simulink model "etherCATmdl2"  (R2022a)
settings: Solver=FixedStepDiscrete  StartTime=0.0  StopTime=inf  RelTol=1e-3
PreLoadFcn:
  | Ts_IO133 = 0.001;
  | Ts_IO750 = 0.001;
InitFcn:
  | Ts_IO133 = 0.001
StopFcn:
  | if isfile(['sdi_view_',bdroot,'.mldatx'])
  |  Simulink.sdi.clearPreferences();
  |  Simulink.sdi.view();
  |  pause(3);
  |  Simulink.sdi.loadView(['sdi_view_',bdroot,]);
  | end
undefined symbols (not defined in the file or in its folder): AUS0, AUS1, C, CAN, FD, padding, Statuswort, Steuerwort
libraries: speedgoatlib_IO602 x9, slrealtimeutilitieslib x8, speedgoatlib_IO133 x5, speedgoatlib_IO750 x5, canfdmsglib x4, canmsglib x4, etargetslib x2, slrealtimeloglib x2, simulink x1
settings Model: SimulationMode=external  ExtModeEnableFloating=off  Creator=sandro.reichenbach  LastModifiedBy=muhammet.cingoez
settings SolverCC: ConcurrentTasks=on  PositivePriorityOrder=on
settings DataIOCC: LimitDataPoints=on  SaveFormat=StructureWithTime
settings OptimizationCC: BlockReduction=off  OptimizeBlockIOStorage=off
settings DebuggingCC: TasksWithSamePriorityMsg=none
settings HardwareCC: ProdBitPerLong=64  ProdLongLongMode=on  ProdHWDeviceType=Intel->x86-64 (Linux 64)
settings RTWCC: Description=Simulink Real-Time  SystemTargetFile=slrealtime.tlc  TemplateMakefile=slrealtime_default_tmf  RTWVerbose=off  Toolchain=Simulink Real-Time Toolchain  BuildConfiguration=Faster Runs  CodeExecutionProfiling=on  TargetLang=C++  DLArmComputeVersion=19.05

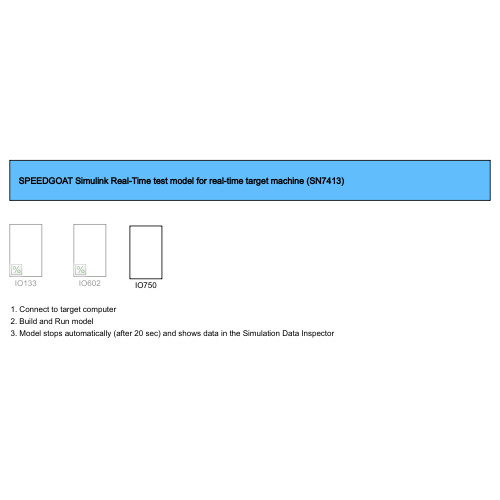
[thumbnail: Simulink's stored preview of the top-level diagram]
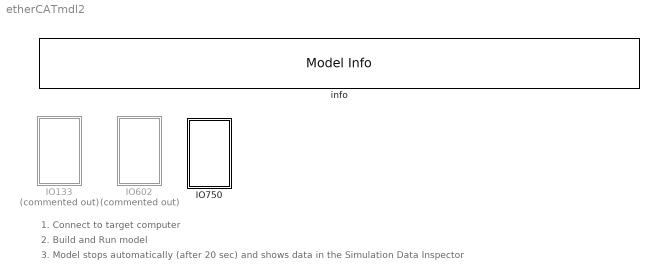
== system etherCATmdl2 ==
  note: 1. Connect to target computer
  note: 2. Build and Run model
  note: 3. Model stops automatically (after 20 sec) and shows data in the Simulation Data Inspector
  IO133 : Subsystem  Commented=on
  IO602 : Subsystem  Commented=on
  IO750 : Subsystem
  info : simulink/Model-Wide Utilities/Model Info  Frame=on  DisplayStringWithTags=SPEEDGOAT Simulink Real-Time test model for real-time target machine (SN7413)  HorizontalTextAlignment=Left  LeftAlignmentValue=0.02

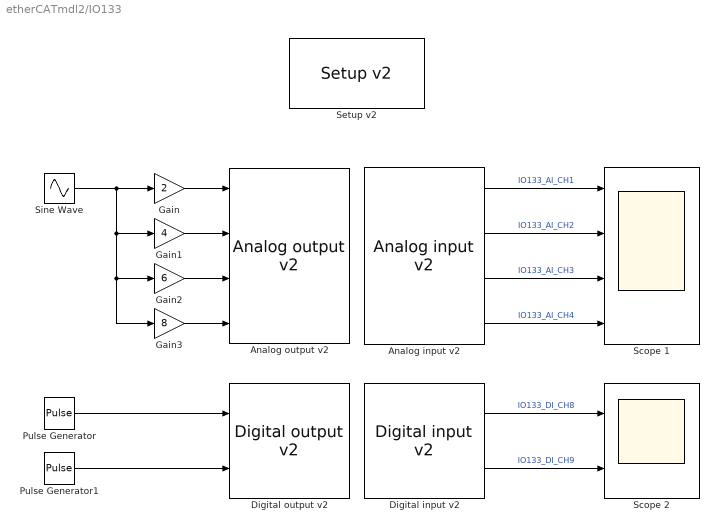
== system etherCATmdl2/IO133 ==
  "Analog input v2 " : speedgoatlib_IO133/Analog input v2   parModuleId=1  parSampleTime=Ts_IO133  parPciSlot=-1  parAdcChannels=[1 2 3 4]  parAdcVoltageRange=[2 2]  parAdcOversamplRate=[1 1]  parAdcContSampling=0  parAdcDmaEnable=0  parAdcActiveDmaDevices=[1 1]  parAdcFrameSize=100
      settings: SourceProductName=Simulink Real-Time: Speedgoat I/O Driver Library
  "Analog output v2 " : speedgoatlib_IO133/Analog output v2   parModuleId=1  parSampleTime=Ts_IO133  parPciSlot=-1  parDacChannels=[1 2 3 4]  parDacVoltageRange=[4 4 6 6 5 5 5 5]  parDacInitValues=[0 0 0 0]  parDacReset=[1 1 1 1]  parDacSyncOut=1  parDacDmaEnable=0  parDacActiveDmaDevices=[1 1]  parDacDmaLatency=2  parDacFrameSize=100
      settings: SourceProductName=Simulink Real-Time: Speedgoat I/O Driver Library
  "Digital input v2 " : speedgoatlib_IO133/Digital input v2   parModuleId=1  parSampleTime=Ts_IO133  parPciSlot=-1  parDiChannels=[8 9]
      settings: SourceProductName=Simulink Real-Time: Speedgoat I/O Driver Library
  "Digital output v2 " : speedgoatlib_IO133/Digital output v2   parModuleId=1  parSampleTime=Ts_IO133  parPciSlot=-1  parDoChannels=[1 2]  parDoInitValues=[0 0]  parDoReset=[1 1]
      settings: SourceProductName=Simulink Real-Time: Speedgoat I/O Driver Library
  Gain : Gain  Gain=2
  Gain1 : Gain  Gain=4
  Gain2 : Gain  Gain=6
  Gain3 : Gain  Gain=8
  Pulse Generator : DiscretePulseGenerator  Period=20  PulseWidth=5  SampleTime=-1
  Pulse Generator1 : DiscretePulseGenerator  Period=20  PulseWidth=10  SampleTime=-1
  Scope 1 : Scope  NumInputPorts=4
  Scope 2 : Scope  NumInputPorts=2
  "Setup v2 " : speedgoatlib_IO133/Setup v2   parPciSlot=-1  parModuleId=1  parInterModuleSync=None  parConvClockBaseRate=20MHz  parConvClock1Divider=20000  parConvClock2Divider=20000  parFrameTriggerEnable=off  parFrameTriggerDivider=10  parConvClock1BaseRate=1  parConvClock2BaseRate=1  parFrameTriggerClock=1  parAdcChannels=1:4  parAdcRange1=+-10V  parAdcRange2=+-10V  parAdcVoltageRange=[2 2]  parAdcOversampling1=None  parAdcOversampling2=None  parAdcOversamplRate=[1 1]  parAdcAutoCorrection=on  parAdcContSampling=off  parAdcDmaEnable=off  parAdcDmaClock=Clock 1  parAdcFrameSize_=100  parAdcSampleTime_=-1  parAdcActiveDmaDevices=[1 1]  parAdcFrameTriggerEnable=0  parAdcFrameSize=100  parAdcSampleTime=0.1  parDacChannels=1:4  parDacInitValues=0  parDacReset=1  parDacRange1=+-5V  parDacRange2=+-5V  parDacRange3=+-10.8V  parDacRange4=+-10.8V  parDacRange5=+-10V  parDacRange6=+-10V  parDacRange7=+-10V  parDacRange8=+-10V  parDacVoltageRange=[4 4 6 6 5 5 5 5]  parDacAutoCorrection=on  parDacSyncOut=on  parDacDmaEnable=off  parDacDmaLatency=Until next frame  parDacDmaClock=Clock 1  parDacFrameSize_=100  parDacSampleTime_=-1  parDacActiveDmaDevices=[1 1]  parDacFrameTriggerEnable=0  parDacFrameSize=100  parDacSampleTime=0.1  parDoChannels=1:2  parDoInitValues=0  parDoReset=1  parDiChannels=8:9  parDiDebounceEnable=off  parDiDebounceTime=0  parDiDebounceValue=0  parDioPullRefFront=Pull-up 3.3V  parDioPullRefRear=Floating
      settings: SourceProductName=Simulink Real-Time: Speedgoat I/O Driver Library
  Sine Wave : Sin  Frequency=50  SampleTime=0
  wires:
  Pulse Generator/1 -> "Digital output v2 "/1
  Gain1/1 -> "Analog output v2 "/2
  Gain/1 -> "Analog output v2 "/1
  Gain3/1 -> "Analog output v2 "/4
  Gain2/1 -> "Analog output v2 "/3
  Sine Wave/1 -> Gain/1, Gain1/1, Gain2/1, Gain3/1
  Pulse Generator1/1 -> "Digital output v2 "/2
  "Analog input v2 "/1 -> Scope 1/1  "IO133_AI_CH1"
  "Analog input v2 "/2 -> Scope 1/2  "IO133_AI_CH2"
  "Analog input v2 "/3 -> Scope 1/3  "IO133_AI_CH3"
  "Analog input v2 "/4 -> Scope 1/4  "IO133_AI_CH4"
  "Digital input v2 "/1 -> Scope 2/1  "IO133_DI_CH8"
  "Digital input v2 "/2 -> Scope 2/2  "IO133_DI_CH9"

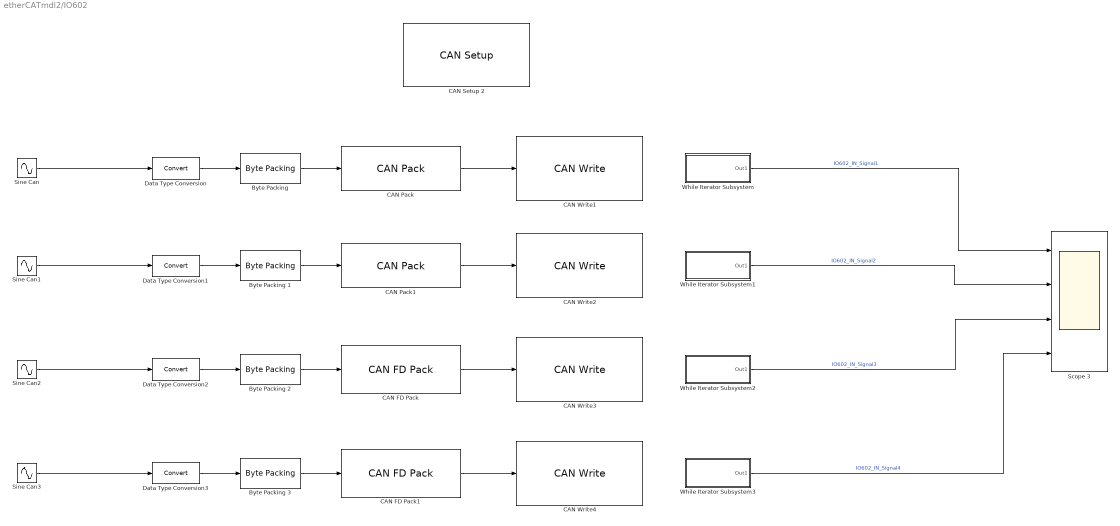
== system etherCATmdl2/IO602 ==
  Byte Packing {,1..3} (4 alike) : slrealtimeutilitieslib/Byte Packing  MaskPackedDataType=uint8  MaskUnpackedDataTypes={'single'}  MaskAlignment=1
  CAN FD Pack : canfdmsglib/CAN FD Pack  MsgList=(none)  MsgName=Msg  ProtocolMode=CAN FD  MsgIDType=Standard (11-bit identifier)  MsgIdentifier=102  MsgLength=4  Remote=off  BRSSwitch=off  ApplyMinMax=off  SignalInfo={}
      settings: SourceProductBaseCode=XP,ME,VN  DataFormat=raw data
  CAN FD Pack1 : canfdmsglib/CAN FD Pack  MsgList=(none)  MsgName=Msg  ProtocolMode=CAN FD  MsgIDType=Standard (11-bit identifier)  MsgIdentifier=103  MsgLength=4  Remote=off  BRSSwitch=off  ApplyMinMax=off  SignalInfo={}
      settings: SourceProductBaseCode=XP,ME,VN  DataFormat=raw data
  CAN Pack : canmsglib/CAN Pack  MsgList=(none)  MsgName=CAN Msg  MsgIDType=Standard (11-bit identifier)  MsgIdentifier=100  MsgLength=4  Remote=off  ApplyMinMax=off  BusOutput=off  SignalInfo={}
      settings: SourceProductBaseCode=XP,ME,VN  DataFormat=raw data
  CAN Pack1 : canmsglib/CAN Pack  MsgList=(none)  MsgName=CAN Msg  MsgIDType=Standard (11-bit identifier)  MsgIdentifier=101  MsgLength=4  Remote=off  ApplyMinMax=off  BusOutput=off  SignalInfo={}
      settings: SourceProductBaseCode=XP,ME,VN  DataFormat=raw data
  CAN Setup 2 : speedgoatlib_IO602/Legacy/CAN Setup   moduletype=IO602  id=1  pciSlot=-1  chn1=CAN (HS)  chn2=CAN (HS)  chn3=CAN-FD  chn4=CAN-FD  initStruct=[]  termStruct=[]  ArbitrationbdrChn1=1.0 MBaud  ArbitrationManbdrChn1=[2,8,31,8]  FdbdrChn1=5.0 MBaud  FdManbdrChn1=[2,2,5,2]  ArbitrationbdrChn2=1.0 MBaud  ArbitrationManbdrChn2=[2,8,31,8]  FdbdrChn2=5.0 MBaud  FdManbdrChn2=[2,2,5,2]  ArbitrationbdrChn3=1.0 MBaud  ArbitrationManbdrChn3=[2,8,31,8]  FdbdrChn3=5.0 MBaud  FdManbdrChn3=[2,2,5,2]  ArbitrationbdrChn4=1.0 MBaud  ArbitrationManbdrChn4=[2,8,31,8]  FdbdrChn4=5.0 MBaud  FdManbdrChn4=[2,2,5,2]  moduleInitValues=[602 1 -1 -1]
      settings: SourceProductName=Simulink Real-Time: Speedgoat I/O Blockset
  CAN Write1 : speedgoatlib_IO602/Legacy/CAN Write  id=1  ts=-1  channel=1  messageType=CAN  BusInput=off  enableStatusPort=off  canType=CAN (HS)  initValues=[602 1 -1 0 1 1 0 0]
      settings: SourceProductName=Simulink Real-Time: Speedgoat I/O Blockset
  CAN Write2 : speedgoatlib_IO602/Legacy/CAN Write  id=1  ts=-1  channel=2  messageType=CAN  BusInput=off  enableStatusPort=off  canType=CAN (HS)  initValues=[602 1 -1 1 1 1 0 0]
      settings: SourceProductName=Simulink Real-Time: Speedgoat I/O Blockset
  CAN Write3 : speedgoatlib_IO602/Legacy/CAN Write  id=1  ts=-1  channel=3  messageType=CAN  BusInput=off  enableStatusPort=off  canType=CAN-FD  initValues=[602 1 -1 2 1 2 0 0]
      settings: SourceProductName=Simulink Real-Time: Speedgoat I/O Blockset
  CAN Write4 : speedgoatlib_IO602/Legacy/CAN Write  id=1  ts=-1  channel=4  messageType=CAN  BusInput=off  enableStatusPort=off  canType=CAN-FD  initValues=[602 1 -1 3 1 2 0 0]
      settings: SourceProductName=Simulink Real-Time: Speedgoat I/O Blockset
  Data Type Conversion{,1..3} (4 alike) : DataTypeConversion  SaturateOnIntegerOverflow=off  RndMeth=Floor
  Scope 3 : Scope  NumInputPorts=4
  Sine Can : Sin  Amplitude=50  Frequency=10*2*pi  SampleTime=0.005
  Sine Can1 : Sin  Amplitude=20  Frequency=10*2*pi  SampleTime=0.005
  Sine Can2 : Sin  Amplitude=30  Frequency=10*2*pi  SampleTime=0.005
  Sine Can3 : Sin  Amplitude=40  Frequency=10*2*pi  SampleTime=0.005
  While Iterator Subsystem : Subsystem  TreatAsAtomicUnit=on
  While Iterator Subsystem1 : Subsystem  TreatAsAtomicUnit=on
  While Iterator Subsystem2 : Subsystem  TreatAsAtomicUnit=on
  While Iterator Subsystem3 : Subsystem  TreatAsAtomicUnit=on
  wires:
  While Iterator Subsystem/1(Out1) -> Scope 3/1  "IO602_IN_Signal1"
  Data Type Conversion/1 -> "Byte Packing "/1
  Sine Can/1 -> Data Type Conversion/1
  CAN Pack/1 -> CAN Write1/1
  "Byte Packing "/1 -> CAN Pack/1
  Byte Packing 1/1 -> CAN Pack1/1
  CAN Pack1/1 -> CAN Write2/1
  Sine Can1/1 -> Data Type Conversion1/1
  Data Type Conversion1/1 -> Byte Packing 1/1
  While Iterator Subsystem1/1(Out1) -> Scope 3/2  "IO602_IN_Signal2"
  While Iterator Subsystem3/1(Out1) -> Scope 3/4  "IO602_IN_Signal4"
  Data Type Conversion3/1 -> Byte Packing 3/1
  Sine Can3/1 -> Data Type Conversion3/1
  CAN FD Pack1/1 -> CAN Write4/1
  Byte Packing 3/1 -> CAN FD Pack1/1
  Byte Packing 2/1 -> CAN FD Pack/1
  CAN FD Pack/1 -> CAN Write3/1
  Sine Can2/1 -> Data Type Conversion2/1
  Data Type Conversion2/1 -> Byte Packing 2/1
  While Iterator Subsystem2/1(Out1) -> Scope 3/3  "IO602_IN_Signal3"

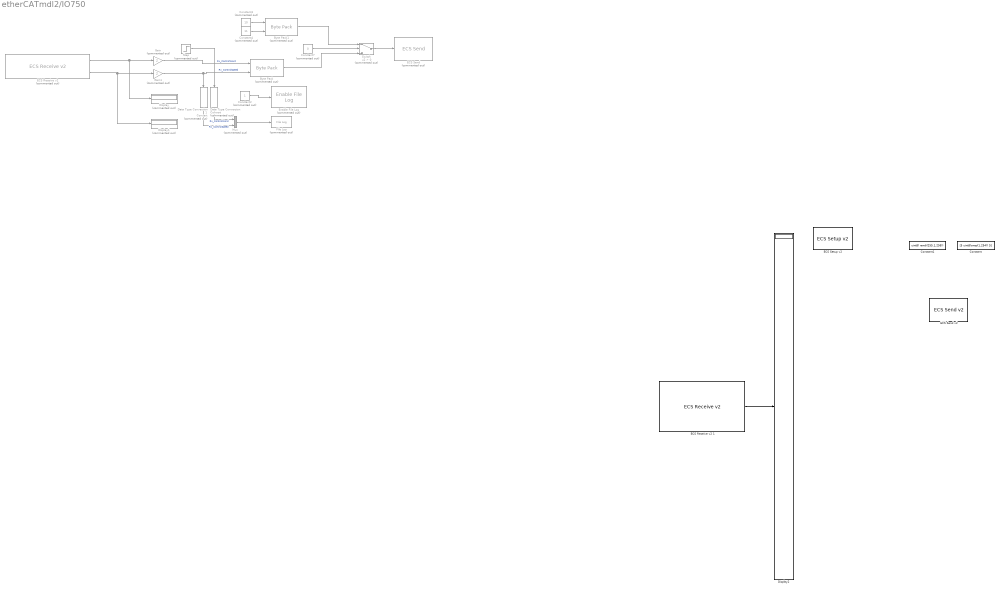
== system etherCATmdl2/IO750 ==
  Byte Pack : etargetslib/Byte Pack  Commented=on  datatypes={'uint32','single'}  byteAlign=1
  Byte Pack1 : etargetslib/Byte Pack  Commented=on  datatypes={'uint32','single'}  byteAlign=1
  Constant : Constant  Value=[5 uint8(ones(1,254)) 5]
  Constant1 : Constant  Value=uint8( randi(255,1,256))
  Constant2 : Constant  Commented=on  OutDataTypeStr=boolean
  Constant3 : Constant  Commented=on  Value=10  OutDataTypeStr=uint32
  Constant4 : Constant  Commented=on  Value=11  OutDataTypeStr=single
  Constant7 : Constant  Commented=on  Value=0  OutDataTypeStr=boolean
  Data Type Conversion : DataTypeConversion  Commented=on  SaturateOnIntegerOverflow=off  RndMeth=Floor
  Data Type Conversion1 : DataTypeConversion  Commented=on  SaturateOnIntegerOverflow=off  RndMeth=Floor
  Display : Display  Commented=on
  Display1 : Display  Commented=on
  Display2 : Display
  "ECS Receive v2 " : speedgoatlib_IO750/ECS Receive v2   Commented=on  id=1  portType=Separate signals  sampleTime=Ts_IO750  pdoTable={ 'Rx', 'ControlWord', 'uint32'; 'Rx', 'ControlSpeed', 'single' }
      settings: SourceProductName=Simulink Real-Time: Speedgoat I/O Blockset
  ECS Receive v2 1 : speedgoatlib_IO750/ECS Receive v2   id=1  portType=Byte vector  sampleTime=Ts_IO750  pdoTable={'Rx1','myvar1','uint8';'Rx2','myvar2','uint8';'Rx3','myvar3','uint8';'Rx4','myvar4','uint8';'Rx5','myvar5','uint8';'Rx6','myvar6','uint8';'Rx7','myvar7','uint8';'Rx8','myvar8','uint8';'Rx9','myvar9','uint8';'Rx10','myvar10','uint8';'Rx11','myvar11','uint8';'Rx12','myvar12','uint8';'Rx13','myvar13','uint8';'Rx14','myvar14','uint8';'Rx15','myvar15','uint8';'Rx16','myvar16','uint8';'Rx17','myvar17','uint8';'Rx18','myvar18','uint8';'Rx19','myvar19','uint8';'Rx20','myvar20','uint8';'Rx21','myvar21','uint8';'Rx22','myvar22','uint8';'Rx23','myvar23','uint8';'Rx24','myvar24','uint8';'Rx25','myvar25','uint8';'Rx26','myvar26','uint8';'Rx27','myvar27','uint8';'Rx28','myvar28','uint8';'Rx29','myvar29','uint8';'Rx30','myvar30','uint8';'Rx31','myvar31','uint8';'Rx32','myvar32','uint8';'Rx33','myvar33','uint8';'Rx34','myvar34','uint8';'Rx35','myvar35','uint8';'Rx36','myvar36','uint8';'Rx37','myvar37','uint8';'Rx38','myvar38','uint8';'Rx39','myvar39','uint8';'Rx40','myvar40','uint8';'Rx41','myvar41','uint8';'Rx42','myvar42','uint8';'Rx43','myvar43','uint8';'Rx44','myvar44','uint8';'Rx45','myvar45','uint8';'Rx46','myvar46','uint8';'Rx47','myvar47','uint8';'Rx48','myvar48','uint8';'Rx49','myvar49','uint8';'Rx50','myvar50','uint8';'Rx51','myvar51','uint8';'Rx52','myvar52','uint8';'Rx53','myvar53','uint8';'Rx54','myvar54','uint8';'Rx55','myvar55','uint8';'Rx56','myvar56','uint8';'Rx57','myvar57','uint8';'Rx58','myvar58','uint8';'Rx59','myvar59','uint8';'Rx60','myvar60','uint8';'Rx61','myvar61','uint8';'Rx62','myvar62','uint8';'Rx63','myvar63','uint8';'Rx64','myvar64','uint8';'Rx65','myvar65','uint8';'Rx66','myvar66','uint8';'Rx67','myvar67','uint8';'Rx68','myvar68','uint8';'Rx69','myvar69','uint8';'Rx70','myvar70','uint8';'Rx71','myvar71','uint8';'Rx72','myvar72','uint8';'Rx73','myvar73','uint8';'Rx74','myvar74','uint8';'Rx75','myvar75','uint8';'Rx76','myvar76','uint8';'Rx77','myvar77','uint8';'Rx78','myvar78','uint8';'Rx79','myvar79','uint8';'Rx80','myvar80','uint8';'Rx81','myvar81','uint8';'Rx82','myvar82','uint8';'Rx83','myvar83','uint8';'Rx84','myvar84','uint8';'Rx85','myvar85','uint8';'Rx86','myvar86','uint8';'Rx87','myvar87','uint8';'Rx88','myvar88','uint8';'Rx89','myvar89','uint8';'Rx90','myvar90','uint8';'Rx91','myvar91','uint8';'Rx92','myvar92','uint8';'Rx93','myvar93','uint8';'Rx94','myvar94','uint8';'Rx95','myvar95','uint8';'Rx96','myvar96','uint8';'Rx97','myvar97','uint8';'Rx98','myvar98','uint8';'Rx99','myvar99','uint8';'Rx100','myvar100','uint8';'Rx101','myvar101','uint8';'Rx102','myvar102','uint8';'Rx103','myvar103','uint8';'Rx104','myvar104','uint8';'Rx105','myvar105','uint8';'Rx106','myvar106','uint8';'Rx107','myvar107','uint8';'Rx108','myvar108','uint8';'Rx109','myvar109','uint8';'Rx110','myvar110','uint8';'Rx111','myvar111','uint8';'Rx112','myvar112','uint8';'Rx113','myvar113','uint8';'Rx114','myvar114','uint8';'Rx115','myvar115','uint8';'Rx116','myvar116','uint8';'Rx117','myvar117','uint8';'Rx118','myvar118','uint8';'Rx119','myvar119','uint8';'Rx120','myvar120','uint8';'Rx121','myvar121','uint8';'Rx122','myvar122','uint8';'Rx123','myvar123','uint8';'Rx124','myvar124','uint8';'Rx125','myvar125','uint8';'Rx126','myvar126','uint8';'Rx127','myvar127','uint8';'Rx128','myvar128','uint8';'Rx129','myvar129','uint8';'Rx130','myvar130','uint8';'Rx131','myvar131','uint8';'Rx132','myvar132','uint8';'Rx133','myvar133','uint8';'Rx134','myvar134','uint8';'Rx135','myvar135','uint8';'Rx136','myvar136','uint8';'Rx137','myvar137','uint8';'Rx138','myvar138','uint8';'Rx139','myvar139','uint8';'Rx140','myvar140','uint8';'Rx141','myvar141','uint8';'Rx142','myvar142','uint8';'Rx143','myvar143','uint8';'Rx144','myvar144','uint8';'Rx145','myvar145','uint8';'Rx146','myvar146','uint8';'Rx147','myvar147','uint8';'Rx148','myvar148','uint8';'Rx149','myvar149','uint8';'Rx150','myvar150','uint8';'Rx151','myvar151','uint8';'Rx152','myvar152','uint8';'Rx153','myvar153','uint8';'Rx154','myvar154','uint8';'Rx155','myvar155','uint8';'Rx156','myvar156','uint8';'Rx157','myvar157','uint8';'Rx158','myvar158','uint8';'Rx159','myvar159','uint8';'Rx160','myvar160','uint8';'Rx161','myvar161','uint8';'Rx162','myvar162','uint8';'Rx163','myvar163','uint8';'Rx164','myvar164','uint8';'Rx165','myvar165','uint8';'Rx166','myvar166','uint8';'Rx167','myvar167','uint8';'Rx168','myvar168','uint8';'Rx169','myvar169','uint8';'Rx170','myvar170','uint8';'Rx171','myvar171','uint8';'Rx172','myvar172','uint8';'Rx173','myvar173','uint8';'Rx174','myvar174','uint8';'Rx175','myvar175','uint8';'Rx176','myvar176','uint8';'Rx177','myvar177','uint8';'Rx178','myvar178','uint8';'Rx179','myvar179','uint8';'Rx180','myvar180','uint8';'Rx181','myvar181','uint8';'Rx182','myvar182','uint8';'Rx183','myvar183','uint8';'Rx184','myvar184','uint8';'Rx185','myvar185','uint8';'Rx186','myvar186','uint8';'Rx187','myvar187','uint8';'Rx188','myvar188','uint8';'Rx189','myvar189','uint8';'Rx190','myvar190','uint8';'Rx191','myvar191','uint8';'Rx192','myvar192','uint8';'Rx193','myvar193','uint8';'Rx194','myvar194','uint8';'Rx195','myvar195','uint8';'Rx196','myvar196','uint8';'Rx197','myvar197','uint8';'Rx198','myvar198','uint8';'Rx199','myvar199','uint8';'Rx200','myvar200','uint8';}
      settings: SourceProductName=Simulink Real-Time: Speedgoat I/O Blockset
  ECS Send : speedgoatlib_IO750/ECS Send  Commented=on  id=1  port_type=1 port with n element vector of type UINT8  out_bytes=8  ts=Ts_IO750
      settings: SourceProductName=Simulink Real-Time: Speedgoat I/O Blockset
  "ECS Send v2 " : speedgoatlib_IO750/ECS Send v2   id=1  portType=Byte vector  sampleTime=-1  pdoTable={'PDO1','myvar1','uint8';'PDO2','myvar2','uint8';'PDO3','myvar3','uint8';'PDO4','myvar4','uint8';'PDO5','myvar5','uint8';'PDO6','myvar6','uint8';'PDO7','myvar7','uint8';'PDO8','myvar8','uint8';'PDO9','myvar9','uint8';'PDO10','myvar10','uint8';'PDO11','myvar11','uint8';'PDO12','myvar12','uint8';'PDO13','myvar13','uint8';'PDO14','myvar14','uint8';'PDO15','myvar15','uint8';'PDO16','myvar16','uint8';'PDO17','myvar17','uint8';'PDO18','myvar18','uint8';'PDO19','myvar19','uint8';'PDO20','myvar20','uint8';'PDO21','myvar21','uint8';'PDO22','myvar22','uint8';'PDO23','myvar23','uint8';'PDO24','myvar24','uint8';'PDO25','myvar25','uint8';'PDO26','myvar26','uint8';'PDO27','myvar27','uint8';'PDO28','myvar28','uint8';'PDO29','myvar29','uint8';'PDO30','myvar30','uint8';'PDO31','myvar31','uint8';'PDO32','myvar32','uint8';'PDO33','myvar33','uint8';'PDO34','myvar34','uint8';'PDO35','myvar35','uint8';'PDO36','myvar36','uint8';'PDO37','myvar37','uint8';'PDO38','myvar38','uint8';'PDO39','myvar39','uint8';'PDO40','myvar40','uint8';'PDO41','myvar41','uint8';'PDO42','myvar42','uint8';'PDO43','myvar43','uint8';'PDO44','myvar44','uint8';'PDO45','myvar45','uint8';'PDO46','myvar46','uint8';'PDO47','myvar47','uint8';'PDO48','myvar48','uint8';'PDO49','myvar49','uint8';'PDO50','myvar50','uint8';'PDO51','myvar51','uint8';'PDO52','myvar52','uint8';'PDO53','myvar53','uint8';'PDO54','myvar54','uint8';'PDO55','myvar55','uint8';'PDO56','myvar56','uint8';'PDO57','myvar57','uint8';'PDO58','myvar58','uint8';'PDO59','myvar59','uint8';'PDO60','myvar60','uint8';'PDO61','myvar61','uint8';'PDO62','myvar62','uint8';'PDO63','myvar63','uint8';'PDO64','myvar64','uint8';'PDO65','myvar65','uint8';'PDO66','myvar66','uint8';'PDO67','myvar67','uint8';'PDO68','myvar68','uint8';'PDO69','myvar69','uint8';'PDO70','myvar70','uint8';'PDO71','myvar71','uint8';'PDO72','myvar72','uint8';'PDO73','myvar73','uint8';'PDO74','myvar74','uint8';'PDO75','myvar75','uint8';'PDO76','myvar76','uint8';'PDO77','myvar77','uint8';'PDO78','myvar78','uint8';'PDO79','myvar79','uint8';'PDO80','myvar80','uint8';'PDO81','myvar81','uint8';'PDO82','myvar82','uint8';'PDO83','myvar83','uint8';'PDO84','myvar84','uint8';'PDO85','myvar85','uint8';'PDO86','myvar86','uint8';'PDO87','myvar87','uint8';'PDO88','myvar88','uint8';'PDO89','myvar89','uint8';'PDO90','myvar90','uint8';'PDO91','myvar91','uint8';'PDO92','myvar92','uint8';'PDO93','myvar93','uint8';'PDO94','myvar94','uint8';'PDO95','myvar95','uint8';'PDO96','myvar96','uint8';'PDO97','myvar97','uint8';'PDO98','myvar98','uint8';'PDO99','myvar99','uint8';'PDO100','myvar100','uint8';'PDO101','myvar101','uint8';'PDO102','myvar102','uint8';'PDO103','myvar103','uint8';'PDO104','myvar104','uint8';'PDO105','myvar105','uint8';'PDO106','myvar106','uint8';'PDO107','myvar107','uint8';'PDO108','myvar108','uint8';'PDO109','myvar109','uint8';'PDO110','myvar110','uint8';'PDO111','myvar111','uint8';'PDO112','myvar112','uint8';'PDO113','myvar113','uint8';'PDO114','myvar114','uint8';'PDO115','myvar115','uint8';'PDO116','myvar116','uint8';'PDO117','myvar117','uint8';'PDO118','myvar118','uint8';'PDO119','myvar119','uint8';'PDO120','myvar120','uint8';'PDO121','myvar121','uint8';'PDO122','myvar122','uint8';'PDO123','myvar123','uint8';'PDO124','myvar124','uint8';'PDO125','myvar125','uint8';'PDO126','myvar126','uint8';'PDO127','myvar127','uint8';'PDO128','myvar128','uint8';'PDO129','myvar129','uint8';'PDO130','myvar130','uint8';'PDO131','myvar131','uint8';'PDO132','myvar132','uint8';'PDO133','myvar133','uint8';'PDO134','myvar134','uint8';'PDO135','myvar135','uint8';'PDO136','myvar136','uint8';'PDO137','myvar137','uint8';'PDO138','myvar138','uint8';'PDO139','myvar139','uint8';'PDO140','myvar140','uint8';'PDO141','myvar141','uint8';'PDO142','myvar142','uint8';'PDO143','myvar143','uint8';'PDO144','myvar144','uint8';'PDO145','myvar145','uint8';'PDO146','myvar146','uint8';'PDO147','myvar147','uint8';'PDO148','myvar148','uint8';'PDO149','myvar149','uint8';'PDO150','myvar150','uint8';'PDO151','myvar151','uint8';'PDO152','myvar152','uint8';'PDO153','myvar153','uint8';'PDO154','myvar154','uint8';'PDO155','myvar155','uint8';'PDO156','myvar156','uint8';'PDO157','myvar157','uint8';'PDO158','myvar158','uint8';'PDO159','myvar159','uint8';'PDO160','myvar160','uint8';'PDO161','myvar161','uint8';'PDO162','myvar162','uint8';'PDO163','myvar163','uint8';'PDO164','myvar164','uint8';'PDO165','myvar165','uint8';'PDO166','myvar166','uint8';'PDO167','myvar167','uint8';'PDO168','myvar168','uint8';'PDO169','myvar169','uint8';'PDO170','myvar170','uint8';'PDO171','myvar171','uint8';'PDO172','myvar172','uint8';'PDO173','myvar173','uint8';'PDO174','myvar174','uint8';'PDO175','myvar175','uint8';'PDO176','myvar176','uint8';'PDO177','myvar177','uint8';'PDO178','myvar178','uint8';'PDO179','myvar179','uint8';'PDO180','myvar180','uint8';'PDO181','myvar181','uint8';'PDO182','myvar182','uint8';'PDO183','myvar183','uint8';'PDO184','myvar184','uint8';'PDO185','myvar185','uint8';'PDO186','myvar186','uint8';'PDO187','myvar187','uint8';'PDO188','myvar188','uint8';'PDO189','myvar189','uint8';'PDO190','myvar190','uint8';'PDO191','myvar191','uint8';'PDO192','myvar192','uint8';'PDO193','myvar193','uint8';'PDO194','myvar194','uint8';'PDO195','myvar195','uint8';'PDO196','myvar196','uint8';'PDO197','myvar197','uint8';'PDO198','myvar198','uint8';'PDO199','myvar199','uint8';'PDO200','myvar200','uint8';}
      settings: SourceProductName=Simulink Real-Time: Speedgoat I/O Blockset
  "ECS Setup v2 " : speedgoatlib_IO750/ECS Setup v2   id=1  drvLetter=C:  configurationMode=Warmstart  busSlot=-1  busStartup=Automatic  dcSync=off  vendorName='Speedgoat'  groupName='Automation'  typeName='IO750'  vendorID=hex2dec('00000001')  productCode=hex2dec('00000002')  revisionNo=hex2dec('00000003')  serialNo=hex2dec('00000004')  stationAlias=0  deviceIdent=0  rxPdoMapping={'Rx1','myvar1','uint8';'Rx2','myvar2','uint8';'Rx3','myvar3','uint8';'Rx4','myvar4','uint8';'Rx5','myvar5','uint8';'Rx6','myvar6','uint8';'Rx7','myvar7','uint8';'Rx8','myvar8','uint8';'Rx9','myvar9','uint8';'Rx10','myvar10','uint8';'Rx11','myvar11','uint8';'Rx12','myvar12','uint8';'Rx13','myvar13','uint8';'Rx14','myvar14','uint8';'Rx15','myvar15','uint8';'Rx16','myvar16','uint8';'Rx17','myvar17','uint8';'Rx18','myvar18','uint8';'Rx19','myvar19','uint8';'Rx20','myvar20','uint8';'Rx21','myvar21','uint8';'Rx22','myvar22','uint8';'Rx23','myvar23','uint8';'Rx24','myvar24','uint8';'Rx25','myvar25','uint8';'Rx26','myvar26','uint8';'Rx27','myvar27','uint8';'Rx28','myvar28','uint8';'Rx29','myvar29','uint8';'Rx30','myvar30','uint8';'Rx31','myvar31','uint8';'Rx32','myvar32','uint8';'Rx33','myvar33','uint8';'Rx34','myvar34','uint8';'Rx35','myvar35','uint8';'Rx36','myvar36','uint8';'Rx37','myvar37','uint8';'Rx38','myvar38','uint8';'Rx39','myvar39','uint8';'Rx40','myvar40','uint8';'Rx41','myvar41','uint8';'Rx42','myvar42','uint8';'Rx43','myvar43','uint8';'Rx44','myvar44','uint8';'Rx45','myvar45','uint8';'Rx46','myvar46','uint8';'Rx47','myvar47','uint8';'Rx48','myvar48','uint8';'Rx49','myvar49','uint8';'Rx50','myvar50','uint8';'Rx51','myvar51','uint8';'Rx52','myvar52','uint8';'Rx53','myvar53','uint8';'Rx54','myvar54','uint8';'Rx55','myvar55','uint8';'Rx56','myvar56','uint8';'Rx57','myvar57','uint8';'Rx58','myvar58','uint8';'Rx59','myvar59','uint8';'Rx60','myvar60','uint8';'Rx61','myvar61','uint8';'Rx62','myvar62','uint8';'Rx63','myvar63','uint8';'Rx64','myvar64','uint8';'Rx65','myvar65','uint8';'Rx66','myvar66','uint8';'Rx67','myvar67','uint8';'Rx68','myvar68','uint8';'Rx69','myvar69','uint8';'Rx70','myvar70','uint8';'Rx71','myvar71','uint8';'Rx72','myvar72','uint8';'Rx73','myvar73','uint8';'Rx74','myvar74','uint8';'Rx75','myvar75','uint8';'Rx76','myvar76','uint8';'Rx77','myvar77','uint8';'Rx78','myvar78','uint8';'Rx79','myvar79','uint8';'Rx80','myvar80','uint8';'Rx81','myvar81','uint8';'Rx82','myvar82','uint8';'Rx83','myvar83','uint8';'Rx84','myvar84','uint8';'Rx85','myvar85','uint8';'Rx86','myvar86','uint8';'Rx87','myvar87','uint8';'Rx88','myvar88','uint8';'Rx89','myvar89','uint8';'Rx90','myvar90','uint8';'Rx91','myvar91','uint8';'Rx92','myvar92','uint8';'Rx93','myvar93','uint8';'Rx94','myvar94','uint8';'Rx95','myvar95','uint8';'Rx96','myvar96','uint8';'Rx97','myvar97','uint8';'Rx98','myvar98','uint8';'Rx99','myvar99','uint8';'Rx100','myvar100','uint8';'Rx101','myvar101','uint8';'Rx102','myvar102','uint8';'Rx103','myvar103','uint8';'Rx104','myvar104','uint8';'Rx105','myvar105','uint8';'Rx106','myvar106','uint8';'Rx107','myvar107','uint8';'Rx108','myvar108','uint8';'Rx109','myvar109','uint8';'Rx110','myvar110','uint8';'Rx111','myvar111','uint8';'Rx112','myvar112','uint8';'Rx113','myvar113','uint8';'Rx114','myvar114','uint8';'Rx115','myvar115','uint8';'Rx116','myvar116','uint8';'Rx117','myvar117','uint8';'Rx118','myvar118','uint8';'Rx119','myvar119','uint8';'Rx120','myvar120','uint8';'Rx121','myvar121','uint8';'Rx122','myvar122','uint8';'Rx123','myvar123','uint8';'Rx124','myvar124','uint8';'Rx125','myvar125','uint8';'Rx126','myvar126','uint8';'Rx127','myvar127','uint8';'Rx128','myvar128','uint8';'Rx129','myvar129','uint8';'Rx130','myvar130','uint8';'Rx131','myvar131','uint8';'Rx132','myvar132','uint8';'Rx133','myvar133','uint8';'Rx134','myvar134','uint8';'Rx135','myvar135','uint8';'Rx136','myvar136','uint8';'Rx137','myvar137','uint8';'Rx138','myvar138','uint8';'Rx139','myvar139','uint8';'Rx140','myvar140','uint8';'Rx141','myvar141','uint8';'Rx142','myvar142','uint8';'Rx143','myvar143','uint8';'Rx144','myvar144','uint8';'Rx145','myvar145','uint8';'Rx146','myvar146','uint8';'Rx147','myvar147','uint8';'Rx148','myvar148','uint8';'Rx149','myvar149','uint8';'Rx150','myvar150','uint8';'Rx151','myvar151','uint8';'Rx152','myvar152','uint8';'Rx153','myvar153','uint8';'Rx154','myvar154','uint8';'Rx155','myvar155','uint8';'Rx156','myvar156','uint8';'Rx157','myvar157','uint8';'Rx158','myvar158','uint8';'Rx159','myvar159','uint8';'Rx160','myvar160','uint8';'Rx161','myvar161','uint8';'Rx162','myvar162','uint8';'Rx163','myvar163','uint8';'Rx164','myvar164','uint8';'Rx165','myvar165','uint8';'Rx166','myvar166','uint8';'Rx167','myvar167','uint8';'Rx168','myvar168','uint8';'Rx169','myvar169','uint8';'Rx170','myvar170','uint8';'Rx171','myvar171','uint8';'Rx172','myvar172','uint8';'Rx173','myvar173','uint8';'Rx174','myvar174','uint8';'Rx175','myvar175','uint8';'Rx176','myvar176','uint8';'Rx177','myvar177','uint8';'Rx178','myvar178','uint8';'Rx179','myvar179','uint8';'Rx180','myvar180','uint8';'Rx181','myvar181','uint8';'Rx182','myvar182','uint8';'Rx183','myvar183','uint8';'Rx184','myvar184','uint8';'Rx185','myvar185','uint8';'Rx186','myvar186','uint8';'Rx187','myvar187','uint8';'Rx188','myvar188','uint8';'Rx189','myvar189','uint8';'Rx190','myvar190','uint8';'Rx191','myvar191','uint8';'Rx192','myvar192','uint8';'Rx193','myvar193','uint8';'Rx194','myvar194','uint8';'Rx195','myvar195','uint8';'Rx196','myvar196','uint8';'Rx197','myvar197','uint8';'Rx198','myvar198','uint8';'Rx199','myvar199','uint8';'Rx200','myvar200','uint8';}  rxPdoCfg=0  rxPdoNames=,Steuerwort,Steuerwort,Statuswort  rxVarNames=,AUS0,padding,AUS1  txPdoMapping={'PDO1','myvar1','uint8';'PDO2','myvar2','uint8';'PDO3','myvar3','uint8';'PDO4','myvar4','uint8';'PDO5','myvar5','uint8';'PDO6','myvar6','uint8';'PDO7','myvar7','uint8';'PDO8','myvar8','uint8';'PDO9','myvar9','uint8';'PDO10','myvar10','uint8';'PDO11','myvar11','uint8';'PDO12','myvar12','uint8';'PDO13','myvar13','uint8';'PDO14','myvar14','uint8';'PDO15','myvar15','uint8';'PDO16','myvar16','uint8';'PDO17','myvar17','uint8';'PDO18','myvar18','uint8';'PDO19','myvar19','uint8';'PDO20','myvar20','uint8';'PDO21','myvar21','uint8';'PDO22','myvar22','uint8';'PDO23','myvar23','uint8';'PDO24','myvar24','uint8';'PDO25','myvar25','uint8';'PDO26','myvar26','uint8';'PDO27','myvar27','uint8';'PDO28','myvar28','uint8';'PDO29','myvar29','uint8';'PDO30','myvar30','uint8';'PDO31','myvar31','uint8';'PDO32','myvar32','uint8';'PDO33','myvar33','uint8';'PDO34','myvar34','uint8';'PDO35','myvar35','uint8';'PDO36','myvar36','uint8';'PDO37','myvar37','uint8';'PDO38','myvar38','uint8';'PDO39','myvar39','uint8';'PDO40','myvar40','uint8';'PDO41','myvar41','uint8';'PDO42','myvar42','uint8';'PDO43','myvar43','uint8';'PDO44','myvar44','uint8';'PDO45','myvar45','uint8';'PDO46','myvar46','uint8';'PDO47','myvar47','uint8';'PDO48','myvar48','uint8';'PDO49','myvar49','uint8';'PDO50','myvar50','uint8';'PDO51','myvar51','uint8';'PDO52','myvar52','uint8';'PDO53','myvar53','uint8';'PDO54','myvar54','uint8';'PDO55','myvar55','uint8';'PDO56','myvar56','uint8';'PDO57','myvar57','uint8';'PDO58','myvar58','uint8';'PDO59','myvar59','uint8';'PDO60','myvar60','uint8';'PDO61','myvar61','uint8';'PDO62','myvar62','uint8';'PDO63','myvar63','uint8';'PDO64','myvar64','uint8';'PDO65','myvar65','uint8';'PDO66','myvar66','uint8';'PDO67','myvar67','uint8';'PDO68','myvar68','uint8';'PDO69','myvar69','uint8';'PDO70','myvar70','uint8';'PDO71','myvar71','uint8';'PDO72','myvar72','uint8';'PDO73','myvar73','uint8';'PDO74','myvar74','uint8';'PDO75','myvar75','uint8';'PDO76','myvar76','uint8';'PDO77','myvar77','uint8';'PDO78','myvar78','uint8';'PDO79','myvar79','uint8';'PDO80','myvar80','uint8';'PDO81','myvar81','uint8';'PDO82','myvar82','uint8';'PDO83','myvar83','uint8';'PDO84','myvar84','uint8';'PDO85','myvar85','uint8';'PDO86','myvar86','uint8';'PDO87','myvar87','uint8';'PDO88','myvar88','uint8';'PDO89','myvar89','uint8';'PDO90','myvar90','uint8';'PDO91','myvar91','uint8';'PDO92','myvar92','uint8';'PDO93','myvar93','uint8';'PDO94','myvar94','uint8';'PDO95','myvar95','uint8';'PDO96','myvar96','uint8';'PDO97','myvar97','uint8';'PDO98','myvar98','uint8';'PDO99','myvar99','uint8';'PDO100','myvar100','uint8';'PDO101','myvar101','uint8';'PDO102','myvar102','uint8';'PDO103','myvar103','uint8';'PDO104','myvar104','uint8';'PDO105','myvar105','uint8';'PDO106','myvar106','uint8';'PDO107','myvar107','uint8';'PDO108','myvar108','uint8';'PDO109','myvar109','uint8';'PDO110','myvar110','uint8';'PDO111','myvar111','uint8';'PDO112','myvar112','uint8';'PDO113','myvar113','uint8';'PDO114','myvar114','uint8';'PDO115','myvar115','uint8';'PDO116','myvar116','uint8';'PDO117','myvar117','uint8';'PDO118','myvar118','uint8';'PDO119','myvar119','uint8';'PDO120','myvar120','uint8';'PDO121','myvar121','uint8';'PDO122','myvar122','uint8';'PDO123','myvar123','uint8';'PDO124','myvar124','uint8';'PDO125','myvar125','uint8';'PDO126','myvar126','uint8';'PDO127','myvar127','uint8';'PDO128','myvar128','uint8';'PDO129','myvar129','uint8';'PDO130','myvar130','uint8';'PDO131','myvar131','uint8';'PDO132','myvar132','uint8';'PDO133','myvar133','uint8';'PDO134','myvar134','uint8';'PDO135','myvar135','uint8';'PDO136','myvar136','uint8';'PDO137','myvar137','uint8';'PDO138','myvar138','uint8';'PDO139','myvar139','uint8';'PDO140','myvar140','uint8';'PDO141','myvar141','uint8';'PDO142','myvar142','uint8';'PDO143','myvar143','uint8';'PDO144','myvar144','uint8';'PDO145','myvar145','uint8';'PDO146','myvar146','uint8';'PDO147','myvar147','uint8';'PDO148','myvar148','uint8';'PDO149','myvar149','uint8';'PDO150','myvar150','uint8';'PDO151','myvar151','uint8';'PDO152','myvar152','uint8';'PDO153','myvar153','uint8';'PDO154','myvar154','uint8';'PDO155','myvar155','uint8';'PDO156','myvar156','uint8';'PDO157','myvar157','uint8';'PDO158','myvar158','uint8';'PDO159','myvar159','uint8';'PDO160','myvar160','uint8';'PDO161','myvar161','uint8';'PDO162','myvar162','uint8';'PDO163','myvar163','uint8';'PDO164','myvar164','uint8';'PDO165','myvar165','uint8';'PDO166','myvar166','uint8';'PDO167','myvar167','uint8';'PDO168','myvar168','uint8';'PDO169','myvar169','uint8';'PDO170','myvar170','uint8';'PDO171','myvar171','uint8';'PDO172','myvar172','uint8';'PDO173','myvar173','uint8';'PDO174','myvar174','uint8';'PDO175','myvar175','uint8';'PDO176','myvar176','uint8';'PDO177','myvar177','uint8';'PDO178','myvar178','uint8';'PDO179','myvar179','uint8';'PDO180','myvar180','uint8';'PDO181','myvar181','uint8';'PDO182','myvar182','uint8';'PDO183','myvar183','uint8';'PDO184','myvar184','uint8';'PDO185','myvar185','uint8';'PDO186','myvar186','uint8';'PDO187','myvar187','uint8';'PDO188','myvar188','uint8';'PDO189','myvar189','uint8';'PDO190','myvar190','uint8';'PDO191','myvar191','uint8';'PDO192','myvar192','uint8';'PDO193','myvar193','uint8';'PDO194','myvar194','uint8';'PDO195','myvar195','uint8';'PDO196','myvar196','uint8';'PDO197','myvar197','uint8';'PDO198','myvar198','uint8';'PDO199','myvar199','uint8';'PDO200','myvar200','uint8';}  txPdoCfg=0  txPdoNames=0  txVarNames=0  sdoMapping={}  sdoCfg=0  sdoNames=0  qtyMods=[1,0,0]  moduleType=IO750  protocol=IO750  firmware=EtherCAT Slave
      settings: SourceProductName=Simulink Real-Time: Speedgoat I/O Blockset
  Enable File Log : slrealtimeloglib/Enable File Log  Commented=on
      settings: SourceProductBaseCode=XP
  File Log : slrealtimeloglib/File Log  Commented=on  decimation=1  inputProcessing=Elements as channels (sample based)
      settings: SourceProductBaseCode=XP
  Gain : Gain  Commented=on  Gain=2  OutDataTypeStr=uint32
  Gain1 : Gain  Commented=on  Gain=2
  Mux : Mux  Commented=on  Inputs=2
  Step : Step  Commented=on  Time=5  Before=2  SampleTime=0.001
  Switch : Switch  Commented=on  Criteria=u2 > Threshold  SaturateOnIntegerOverflow=off  InputSameDT=off
  wires:
  "ECS Receive v2 "/1 -> Display/1, Gain/1
  "ECS Receive v2 "/2 -> Display1/1, Gain1/1
  Gain/1 -> Byte Pack/1  "Rx_ControlWord"
  Gain1/1 -> Data Type Conversion1/1, Byte Pack/2  "Rx_ControlSpeed"
  Constant2/1 -> Enable File Log/1
  Mux/1 -> File Log/1
  Data Type Conversion/1 -> Mux/1  "Rx_ControlWord"
  Data Type Conversion1/1 -> Mux/2  "Rx_ControlSpeed"
  Step/1 -> Data Type Conversion/1
  Constant3/1 -> Byte Pack1/1
  Constant4/1 -> Byte Pack1/2
  Switch/1 -> ECS Send/1
  Byte Pack1/1 -> Switch/1
  Byte Pack/1 -> Switch/3
  Constant7/1 -> Switch/2
  ECS Receive v2 1/1 -> Display2/1

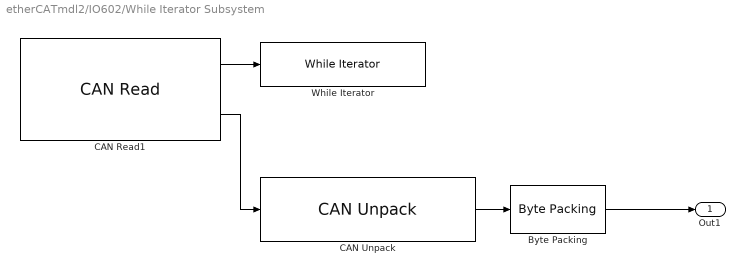
== system etherCATmdl2/IO602/While Iterator Subsystem ==
  "Byte Packing " : slrealtimeutilitieslib/Byte Packing  MaskPackedDataType=single  MaskUnpackedDataTypes={'uint8'}  MaskAlignment=1
  CAN Read1 : speedgoatlib_IO602/Legacy/CAN Read  id=1  ts=-1  channel=1  messageType=CAN  canType=CAN (HS)  BusOutput=off  initValues=[602 1 -1 0 1 1 0]
      settings: SourceProductName=Simulink Real-Time: Speedgoat I/O Blockset
  CAN Unpack : canmsglib/CAN Unpack  MsgList=(none)  MsgName=CAN Msg  MsgIDType=Standard (11-bit identifier)  MsgIdentifier=101  MsgLength=4  SignalInfo={}  IDPort=off  TimestampPort=off  ErrorPort=off  RemotePort=off  LengthPort=off  StatusPort=off  ApplyMinMax=off
      settings: SourceProductBaseCode=XP,ME,VN  DataFormat=raw data
  While Iterator : WhileIterator  MaxIters=50  WhileBlockType=do-while
  Out1 : Outport
  wires:
  "Byte Packing "/1 -> Out1/1
  CAN Unpack/1 -> "Byte Packing "/1
  CAN Read1/2 -> CAN Unpack/1
  CAN Read1/1 -> While Iterator/1

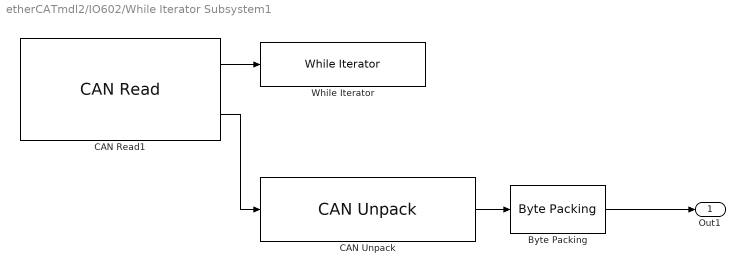
== system etherCATmdl2/IO602/While Iterator Subsystem1 ==
  "Byte Packing " : slrealtimeutilitieslib/Byte Packing  MaskPackedDataType=single  MaskUnpackedDataTypes={'uint8'}  MaskAlignment=1
  CAN Read1 : speedgoatlib_IO602/Legacy/CAN Read  id=1  ts=-1  channel=2  messageType=CAN  canType=CAN (HS)  BusOutput=off  initValues=[602 1 -1 1 1 1 0]
      settings: SourceProductName=Simulink Real-Time: Speedgoat I/O Blockset
  CAN Unpack : canmsglib/CAN Unpack  MsgList=(none)  MsgName=CAN Msg  MsgIDType=Standard (11-bit identifier)  MsgIdentifier=100  MsgLength=4  SignalInfo={}  IDPort=off  TimestampPort=off  ErrorPort=off  RemotePort=off  LengthPort=off  StatusPort=off  ApplyMinMax=off
      settings: SourceProductBaseCode=XP,ME,VN  DataFormat=raw data
  While Iterator : WhileIterator  MaxIters=50  WhileBlockType=do-while
  Out1 : Outport
  wires:
  CAN Read1/1 -> While Iterator/1
  CAN Read1/2 -> CAN Unpack/1
  CAN Unpack/1 -> "Byte Packing "/1
  "Byte Packing "/1 -> Out1/1

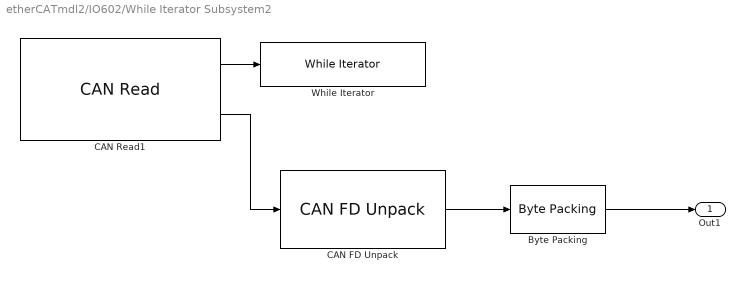
== system etherCATmdl2/IO602/While Iterator Subsystem2 ==
  "Byte Packing " : slrealtimeutilitieslib/Byte Packing  MaskPackedDataType=single  MaskUnpackedDataTypes={'uint8'}  MaskAlignment=1
  CAN FD Unpack : canfdmsglib/CAN FD Unpack  MsgList=(none)  MsgName=Msg  ProtocolMode=CAN FD  MsgIDType=Standard (11-bit identifier)  MsgIdentifier=103  MsgLength=4  SignalInfo={}  IDPort=off  TimestampPort=off  ErrorPort=off  RemotePort=off  LengthPort=off  StatusPort=off  BRSPort=off  ESIPort=off  DLCPort=off  ApplyMinMax=off
      settings: SourceProductBaseCode=XP,ME,VN  DataFormat=raw data
  CAN Read1 : speedgoatlib_IO602/Legacy/CAN Read  id=1  ts=-1  channel=3  messageType=CAN  canType=CAN-FD  BusOutput=off  initValues=[602 1 -1 2 1 2 0]
      settings: SourceProductName=Simulink Real-Time: Speedgoat I/O Blockset
  While Iterator : WhileIterator  MaxIters=50  WhileBlockType=do-while
  Out1 : Outport
  wires:
  CAN Read1/1 -> While Iterator/1
  CAN Read1/2 -> CAN FD Unpack/1
  CAN FD Unpack/1 -> "Byte Packing "/1
  "Byte Packing "/1 -> Out1/1

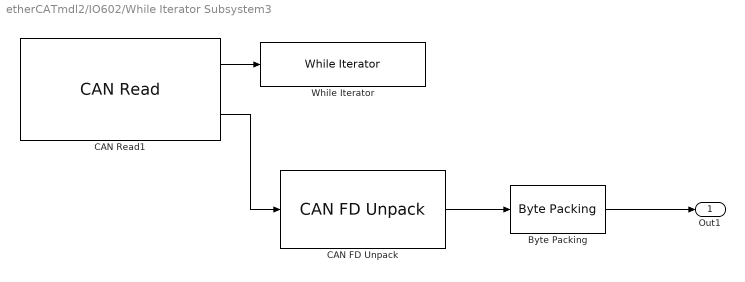
== system etherCATmdl2/IO602/While Iterator Subsystem3 ==
  "Byte Packing " : slrealtimeutilitieslib/Byte Packing  MaskPackedDataType=single  MaskUnpackedDataTypes={'uint8'}  MaskAlignment=1
  CAN FD Unpack : canfdmsglib/CAN FD Unpack  MsgList=(none)  MsgName=Msg  ProtocolMode=CAN FD  MsgIDType=Standard (11-bit identifier)  MsgIdentifier=102  MsgLength=4  SignalInfo={}  IDPort=off  TimestampPort=off  ErrorPort=off  RemotePort=off  LengthPort=off  StatusPort=off  BRSPort=off  ESIPort=off  DLCPort=off  ApplyMinMax=off
      settings: SourceProductBaseCode=XP,ME,VN  DataFormat=raw data
  CAN Read1 : speedgoatlib_IO602/Legacy/CAN Read  id=1  ts=-1  channel=4  messageType=CAN  canType=CAN-FD  BusOutput=off  initValues=[602 1 -1 3 1 2 0]
      settings: SourceProductName=Simulink Real-Time: Speedgoat I/O Blockset
  While Iterator : WhileIterator  MaxIters=50  WhileBlockType=do-while
  Out1 : Outport
  wires:
  "Byte Packing "/1 -> Out1/1
  CAN FD Unpack/1 -> "Byte Packing "/1
  CAN Read1/2 -> CAN FD Unpack/1
  CAN Read1/1 -> While Iterator/1
